simulink model "DSSS_tranmission chain spectrum analysis"  (R2016a)
settings: Solver=VariableStepAuto  StartTime=0.0  StopTime=2  RelTol=1e-3
libraries: dspfdesign x2, commutil2 x2, commblkcod2 x1, commblkintrlv2 x1, commseqgen3 x1, commrandsrc3 x1, commsequence2 x1
settings Model: Creator=malaika  LastModifiedBy=malaika

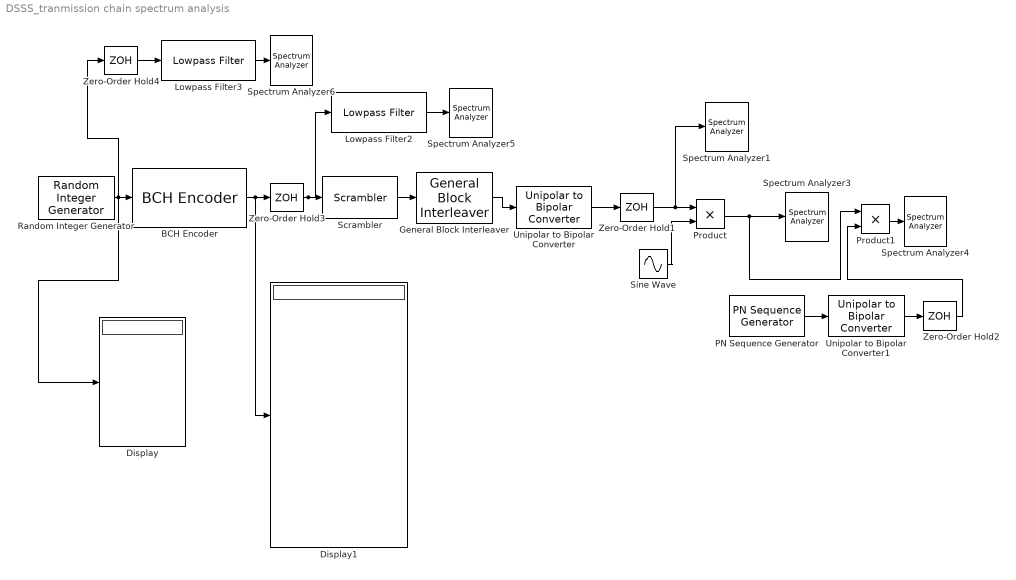
== system DSSS_tranmission chain spectrum analysis ==
  BCH Encoder : commblkcod2/BCH Encoder  n=15  k=5  specShortening=off  shortenedK=5  specGenPoly=off  genPoly='X^10 + X^8 + X^5 + X^4 + X^2 + X + 1'  specPrimPoly=off  prPoly='X^4 + X + 1'  specDisableGenCheck=off  specPuncture=off  punctVec=[ones(8,1); zeros(2,1)]
  Display : Display
  Display1 : Display
  General Block Interleaver : commblkintrlv2/General Block Interleaver  permutationVectorSource=Dialog  elements=[15:-1:1].'
  Lowpass Filter2 : dspfdesign/Lowpass Filter  FilterType=FIR  DesignForMinimumOrder=on  FilterOrder=50  PassbandFrequency=1400  StopbandFrequency=1500  PassbandRipple=0.1  StopbandAttenuation=80  InheritSampleRate=on  SampleRate=44100  roundingMode=Floor  coeffsDataTypeStr=fixdt(1,16)  SimulateUsing=Interpreted execution
  Lowpass Filter3 : dspfdesign/Lowpass Filter  FilterType=FIR  DesignForMinimumOrder=on  FilterOrder=50  PassbandFrequency=400  StopbandFrequency=500  PassbandRipple=0.1  StopbandAttenuation=80  InheritSampleRate=on  SampleRate=44100  roundingMode=Floor  coeffsDataTypeStr=fixdt(1,16)  SimulateUsing=Interpreted execution
  PN Sequence Generator : commseqgen3/PN Sequence Generator  poly='z^10 + z^3 + 1'  ini_sta=[0 0 0 0 0 0 0 0 0 1]  outBitMaskSource=Dialog parameter  shift=0  outVarSiz=off  maxOutSizeMode=Dialog parameter  maxOutSize=[10 1]  Ts=1/15000  sampPerFrame=1  reset=off  bitPackedOutputs=off  outDataType=double  numPackedBits=8  bitPackDataSigned=off  bitPackedOutDType=double
  Product : Product
  Product1 : Product
  Random Integer Generator : commrandsrc3/Random Integer Generator  SetSize=2  SeedSource=Auto  Seed=0  SampleTime=0.002  SamplesPerFrame=5  OutputDataType=double  SimulateUsing=Interpreted execution
  Scrambler : commsequence2/Scrambler  M=2  poly='1 + z^-1 + z^-2 + z^-4'  iniStaSource=Dialog Parameter  ini_sta=[0 1 0 1]  resetViaPort=off
  Sine Wave : Sin  Frequency=2*pi*5000  SampleTime=0.00002
  Spectrum Analyzer{1,3..6} (5 alike) : SpectrumAnalyzer
  Unipolar to Bipolar Converter : commutil2/Unipolar to Bipolar Converter  M=2  polarity=Positive  dataType=Inherit via internal rule
  Unipolar to Bipolar Converter1 : commutil2/Unipolar to Bipolar Converter  M=2  polarity=Positive  dataType=Inherit via internal rule
  Zero-Order Hold1 : ZeroOrderHold  SampleTime=0.00002
  Zero-Order Hold2 : ZeroOrderHold  SampleTime=0.00002
  Zero-Order Hold3 : ZeroOrderHold  SampleTime=0.0006667
  Zero-Order Hold4 : ZeroOrderHold  SampleTime=0.002/3
  wires:
  Unipolar to Bipolar Converter/1 -> Zero-Order Hold1/1
  Zero-Order Hold1/1 -> Spectrum Analyzer1/1, Product/1
  Sine Wave/1 -> Product/2
  Product/1 -> Product1/1, Spectrum Analyzer3/1
  PN Sequence Generator/1 -> Unipolar to Bipolar Converter1/1
  Zero-Order Hold2/1 -> Product1/2
  Product1/1 -> Spectrum Analyzer4/1
  BCH Encoder/1 -> Display1/1, Zero-Order Hold3/1
  Unipolar to Bipolar Converter1/1 -> Zero-Order Hold2/1
  Scrambler/1 -> General Block Interleaver/1
  General Block Interleaver/1 -> Unipolar to Bipolar Converter/1
  Lowpass Filter2/1 -> Spectrum Analyzer5/1
  Zero-Order Hold4/1 -> Lowpass Filter3/1
  Lowpass Filter3/1 -> Spectrum Analyzer6/1
  Random Integer Generator/1 -> Display/1, Zero-Order Hold4/1, BCH Encoder/1
  Zero-Order Hold3/1 -> Lowpass Filter2/1, Scrambler/1
